simulink model "DroneModel"  (R2020a)
settings: Solver=VariableStepAuto  StartTime=0.0  StopTime=100  RelTol=1e-3
libraries: simulink x1
settings Model: Creator=rjvar  LastModifiedBy=rjvar

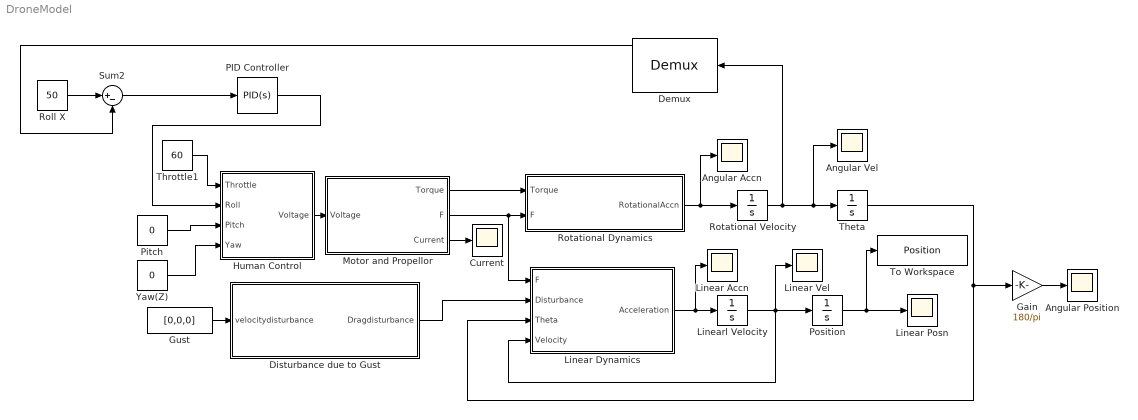
== system DroneModel ==
  Angular Accn : Scope
  Angular Position : Scope
  Angular Vel : Scope
  Current : Scope
  Demux : Demux  Outputs=3
  Disturbance due to Gust : MATLAB Function  TreatAsAtomicUnit=on
  Gain : Gain  Gain=180/pi
  Gust : Constant  Value=[0,0,0]
  Human Control : MATLAB Function  TreatAsAtomicUnit=on
  Linear Accn : Scope
  Linear Dynamics : MATLAB Function  TreatAsAtomicUnit=on
  Linear Posn : Scope
  Linear Vel : Scope
  Linearl Velocity : Integrator
  Motor and Propellor : MATLAB Function  TreatAsAtomicUnit=on
  PID Controller : simulink/Continuous/PID Controller  Controller=PID  Form=Parallel  TimeDomain=Continuous-time  UseExternalTs=off  SampleTime=-1  IntegratorMethod=Forward Euler  FilterMethod=Forward Euler  ControllerParametersSource=internal  P=7.212  I=13.924  D=-0.197  UseFilter=on  N=100  TunerSelectOption=Transfer Function Based (PID Tuner App)  InitialConditionSource=internal  InitialConditionForIntegrator=0  InitialConditionForFilter=0  DifferentiatorICPrevScaledInput=0  ExternalReset=none  TrackingMode=off  Kt=1  LimitOutput=on  UpperSaturationLimit=100  LowerSaturationLimit=0  LinearizeAsGain=on  AntiWindupMode=clamping  Kb=1  POutMin=[]  POutMax=[]  IOutMin=[]  IOutMax=[]  DOutMin=[]  DOutMax=[]  NOutMin=[]  NOutMax=[]  SumOutMin=[]  SumOutMax=[]  SaturationOutMin=[]  SaturationOutMax=[]  PParamMin=[]  PParamMax=[]  IParamMin=[]  IParamMax=[]  DParamMin=[]  DParamMax=[]  NParamMin=[]  NParamMax=[]  KbParamMin=[]  KbParamMax=[]  KtParamMin=[]  KtParamMax=[]  KbOutMin=[]  KbOutMax=[]  KtOutMin=[]  KtOutMax=[]  IntegratorOutMin=[]  IntegratorOutMax=[]  FilterOutMin=[]  FilterOutMax=[]  SumI1OutMin=[]  SumI1OutMax=[]  SumI2OutMin=[]  SumI2OutMax=[]  SumI3OutMin=[]  SumI3OutMax=[]  SumI4OutMin=[]  SumI4OutMax=[]  SumDOutMin=[]  SumDOutMax=[]  DifferentiatorOutMin=[]  DifferentiatorOutMax=[]  FilterDiffOutCoefMin=[]  FilterDiffOutCoefMax=[]  ReciprocalOutMin=[]  ReciprocalOutMax=[]  SumDenOutMin=[]  SumDenOutMax=[]  SumNumOutMin=[]  SumNumOutMax=[]  DivideOutMin=[]  DivideOutMax=[]  UdiffTsProdOutMin=[]  UdiffTsProdOutMax=[]  NTsProdOutMin=[]  NTsProdOutMax=[]  UintegralTsProdOutMin=[]  UintegralTsProdOutMax=[]  UngainTsProdOutMin=[]  UngainTsProdOutMax=[]  IntegratorContinuousStateAttributes=''  IntegratorStateMustResolveToSignalObject=off  IntegratorRTWStateStorageClass=Auto  FilterContinuousStateAttributes=''  FilterStateMustResolveToSignalObject=off  FilterRTWStateStorageClass=Auto  ParallelPVariant=InternalParameters  IdealPVariant=Disabled  IVariant=InternalParameters  DVariant=InternalParameters  IntegratorVariant=Continuous  SatVariant=Enabled  AWVariant=ContClampingParallel  PCopyVariant=Disabled  TRVariant=Disabled  FdbkBlocksVariant=Forward  IdealPFdbkVariant=Disabled  SatFdbkVariant=Disabled  DerivativeFilterVariant=ContFilter  NVariant=InternalParameters  NCopyVariant=Disabled  FilterICVariant=InternalICsFilter  IntegratorICVariant=InternalICs  ExternalResetVariant=Disabled  TRSumVariant=Passthrough  SumFdbkVariant=Disabled  SumVariant=Sum_PID  TsampFilterVariant=InternalTs  TsampNgainVariant=Passthrough  TsampIntegralVariant=Passthrough
  Pitch : Constant  Value=0
  Position : Integrator
  Roll X : Constant  Value=50
  Rotational Dynamics : MATLAB Function  TreatAsAtomicUnit=on
  Rotational Velocity : Integrator
  Sum2 : Sum  Inputs=|+-
  Theta : Integrator
  Throttle1 : Constant  Value=60
  To Workspace : ToWorkspace  VariableName=Position  SampleTime=-1
      settings: Save2DSignal=2-D array (concatenate along first dimension)
  Yaw(Z) : Constant  Value=0
  wires:
  Motor and Propellor/2(F) -> Linear Dynamics/1(F), Rotational Dynamics/2(F)
  Motor and Propellor/1(Torque) -> Rotational Dynamics/1(Torque)
  Rotational Dynamics/1(RotationalAccn) -> Rotational Velocity/1, Angular Accn/1
  Theta/1 -> Linear Dynamics/3(Theta), Gain/1
  Linear Dynamics/1(Acceleration) -> Linear Accn/1, Linearl Velocity/1
  Linearl Velocity/1 -> Linear Dynamics/4(Velocity), Linear Vel/1, Position/1
  Disturbance due to Gust/1(Dragdisturbance) -> Linear Dynamics/2(Disturbance)
  Gust/1 -> Disturbance due to Gust/1(velocitydisturbance)
  Human Control/1(Voltage) -> Motor and Propellor/1(Voltage)
  Yaw(Z)/1 -> Human Control/4(Yaw)
  Gain/1 -> Angular Position/1
  Motor and Propellor/3(Current) -> Current/1
  Position/1 -> Linear Posn/1, To Workspace/1
  Sum2/1 -> PID Controller/1
  Roll X/1 -> Sum2/1
  Pitch/1 -> Human Control/3(Pitch)
  Rotational Velocity/1 -> Demux/1, Theta/1, Angular Vel/1
  PID Controller/1 -> Human Control/2(Roll)
  Throttle1/1 -> Human Control/1(Throttle)
  Demux/1 -> Sum2/2

== matlab function DroneModel/Rotational Dynamics ==
  data: Torque input; RotationalAccn output; F input
function RotationalAccn = fcn(Torque,F)
Moment = [0,0,0];
RotationalAccn = [0,0,0];
I = [0.003,0.003,0.007];
Moment(1) = (F(3)+F(4))*(0.237/2)-(F(1)+F(2))*(0.237/2);
Moment(2) = (F(3)+F(2))*(0.237/2)-(F(1)+F(4))*(0.237/2);
Moment(3) = Torque(4)-Torque(1)+Torque(2)-Torque(3);
for i=1:3
    RotationalAccn(i) = Moment(i)/I(i);
end

== matlab function DroneModel/Motor and Propellor ==
  data: Voltage input; Torque output; F output; Current output
function [Torque,F,Current] = fcn(Voltage)
RPM = [0,0,0,0];
Torque = [0,0,0,0];
Current = [0,0,0,0];
F = [0,0,0,0];
for i=1:4
    RPM(i) = -2.6931*Voltage(i)^3+1400*Voltage(i);
    Ct = 2*10^-15*RPM(i)^3 -4*10^-11*RPM(i)^2+3*10^-7*RPM(i)+0.1013;
    F(i) = Ct*1.225*(RPM(i)/60)^2*0.2^4;
    Torque(i) = 4*10^-14*RPM(i)^3+8*10^-12*RPM(i)^2+3*10^-6*RPM(i);
    Current(i) = 1400*Torque(i);
end

== matlab function DroneModel/Linear Dynamics ==
  data: F input; Acceleration output; Disturbance input; Theta input; Velocity input
function Acceleration = fcn(F,Disturbance,Theta,Velocity)
m=0.743;
g = 9.81;
A = [0.0197,0.0197,0.0512];%Projected Area
rho = 1.225;
Cd = 1;%insert actual Drag coefficient 
Acceleration = [0 0 0];
Force = [0 0 0];
Fprop = [0 0 0];
Fprop(1) = sin(Theta(2))*cos(Theta(1))*(F(1)+F(2)+F(3)+F(4)); %Force created by propellor in x direction
Fprop(2) = sin(Theta(1))*cos(Theta(2))*(F(1)+F(2)+F(3)+F(4)); %Force created by propellor in y direction
Fprop(3) = cos(Theta(1))*cos(Theta(2))*(F(1)+F(2)+F(3)+F(4)); %Force created by propellor in z direction
ThetaXY = -atan2(Fprop(1),Fprop(2));
XY2D = sqrt(Fprop(1)^2 + Fprop(2)^2);
if Fprop(3)>=0
    Fprop(1) = XY2D*sin(ThetaXY+Theta(3));
    Fprop(2) = XY2D*cos(ThetaXY+Theta(3));
else
    Fprop(1) = XY2D*sin(ThetaXY-Theta(3));
    Fprop(2) = XY2D*cos(ThetaXY-Theta(3));
end
if Velocity(1)<0
    Force(1) = Fprop(1)-Disturbance(1)+0.5*rho*Velocity(1)^2*A(1)*Cd;
else
    Force(1) = Fprop(1)-Disturbance(1)-0.5*rho*Velocity(1)^2*A(1)*Cd;
end
if Velocity(2)<0
    Force(2) = Fprop(2)-Disturbance(2)+0.5*rho*Velocity(2)^2*A(2)*Cd;
else
    Force(2) = Fprop(2)-Disturbance(2)-0.5*rho*Velocity(2)^2*A(2)*Cd;
end
if Velocity(3)<0
    Force(3) = Fprop(3)-Disturbance(3)+0.5*rho*Velocity(3)^2*A(3)*Cd-m*g;
else
    Force(3) = Fprop(3)-Disturbance(3)-0.5*rho*Velocity(3)^2*A(3)*Cd-m*g;
end
for i=1:3
    Acceleration(i) = Force(i)/m;
end

== matlab function DroneModel/Disturbance due to Gust ==
  data: velocitydisturbance input; Dragdisturbance output
function Dragdisturbance = fcn(velocitydisturbance)
A = [0.0197 0.0197 0.0197*2*1.3];
Dragdisturbance = [0 0 0];
rho = 1.225;
Cd = 1;
%Direction of gust
for i=1:3
    if velocitydisturbance(i)<0
        Dragdisturbance(i) = 0.5*Cd*rho*A(i)*(velocitydisturbance(i))^2;
    else
        Dragdisturbance(i) = -0.5*Cd*rho*A(i)*(velocitydisturbance(i))^2;
    end
end

== matlab function DroneModel/Human Control ==
  data: Throttle input; Voltage output; Roll input; Pitch input; Yaw input
function Voltage = fcn(Throttle, Roll, Pitch, Yaw)
Correct = 0;
if (Pitch/2+Roll/2+Yaw/2)>(100-Throttle)
    Correct = (Pitch/2+Roll/2+Yaw/2)-(100-Throttle);
end
if (Pitch/2+Roll/2+Yaw/2)>(Throttle)
    if Correct<((Pitch/2+Roll/2+Yaw/2)-(Throttle))
        Correct = (Pitch/2+Roll/2+Yaw/2)-(Throttle);
    end
end
if Correct~=0
    Pitch = Pitch-Correct/3*2;
    Roll = Roll-Correct/3*2;
    Yaw = Yaw-Correct/3*2;
end
Voltage = [(Throttle-Pitch/2-Roll/2-Yaw/2)*11.4/100 (Throttle-Pitch/2+Roll/2+Yaw/2)*11.4/100 (Throttle+Pitch/2+Roll/2-Yaw/2)*11.4/100 (Throttle+Pitch/2-Roll/2+Yaw/2)*11.4/100];    



%If we want Roll pitch and Yaw , then we are subtracting left throttle with
%Roll Pithc an Yaw, that we want to apply,we can increase 50% throttle on 1
%side and decrease 50% throttle on other side
%correct tells what is the excess power that we can apply to give roll
%pitch and yaw
